simulink model "Two_Zone_MVDC_PSolver_Thermal_R2020b"  (R2020b)
settings: Solver=FixedStepDiscrete  StartTime=0.0  StopTime=30  FixedStep=TsELEC  RelTol=1e-3  EnableMultiTasking=on
InitFcn:
  | TsELEC = 25e-6;
  | Ts = 25e-6;
  | TsTHERMAL = 1e-3;
  | TsCont = TsELEC;
  | Rsnub = 1e4;
undefined symbols (not defined in the file or in its folder): DiscIntNeverNeededParam, ee_sli_rtmsupport, GABDA, GABDB, GBBDA, GBBDB, gcbh, GPMMA, GPPMB, GPPMC, SADA, SADB, SADC, SADD, SBDA, SBDB, SBDC, SCDA, SCDB, SCDC, SCDD, SDDA, SDDB, SDDC, SDDD, SDDE
libraries: fl_lib x201, nesl_utility x93, ee_lib x52, SimscapeFluids_lib x4, simulink x3, pid_lib x3, eeTransforms x3, sps_avr x2, powerlib_meascontrol x2, slrealtimetgmanagement x1
(part 5 of 5)

== system Two_Zone_MVDC_PSolver_Thermal_R2020b/Subsystem3/Control/Torque Control/Control_System/Current_Controllers/PI_Controller_Id ==
  I_ref : Inport
  I_fb : Inport  Port=2
  Constant : Constant  Value=0  SampleTime=TsELEC
  Discrete PID Controller : pid_lib/PID Controller  Controller=PID  Form=Parallel  TimeDomain=Discrete-time  UseExternalTs=off  SampleTime=TsELEC  IntegratorMethod=Forward Euler  FilterMethod=Forward Euler  ControllerParametersSource=internal  P=2/10  I=340/10  D=0  UseFilter=on  N=100  TunerSelectOption=Transfer Function Based (PID Tuner App)  InitialConditionSource=internal  InitialConditionForIntegrator=0  InitialConditionForFilter=0  DifferentiatorICPrevScaledInput=0  ExternalReset=either  TrackingMode=off  Kt=1  LimitOutput=off  SatLimitsSource=internal  UpperSaturationLimit=inf  LowerSaturationLimit=-inf  LinearizeAsGain=off  AntiWindupMode=none  Kb=1  POutMin=[]  POutMax=[]  IOutMin=[]  IOutMax=[]  DOutMin=[]  DOutMax=[]  NOutMin=[]  NOutMax=[]  SumOutMin=[]  SumOutMax=[]  SaturationOutMin=[]  SaturationOutMax=[]  PParamMin=[]  PParamMax=[]  IParamMin=[]  IParamMax=[]  DParamMin=[]  DParamMax=[]  NParamMin=[]  NParamMax=[]  KbParamMin=[]  KbParamMax=[]  KtParamMin=[]  KtParamMax=[]  KbOutMin=[]  KbOutMax=[]  KtOutMin=[]  KtOutMax=[]  IntegratorOutMin=[]  IntegratorOutMax=[]  FilterOutMin=[]  FilterOutMax=[]  SumI1OutMin=[]  SumI1OutMax=[]  SumI2OutMin=[]  SumI2OutMax=[]  SumI3OutMin=[]  SumI3OutMax=[]  SumI4OutMin=[]  SumI4OutMax=[]  SumDOutMin=[]  SumDOutMax=[]  DifferentiatorOutMin=[]  DifferentiatorOutMax=[]  FilterDiffOutCoefMin=[]  FilterDiffOutCoefMax=[]  ReciprocalOutMin=[]  ReciprocalOutMax=[]  SumDenOutMin=[]  SumDenOutMax=[]  SumNumOutMin=[]  SumNumOutMax=[]  DivideOutMin=[]  DivideOutMax=[]  UdiffTsProdOutMin=[]  UdiffTsProdOutMax=[]  NTsProdOutMin=[]  NTsProdOutMax=[]  UintegralTsProdOutMin=[]  UintegralTsProdOutMax=[]  UngainTsProdOutMin=[]  UngainTsProdOutMax=[]  IntegratorContinuousStateAttributes=''  IntegratorStateMustResolveToSignalObject=off  IntegratorRTWStateStorageClass=Auto  FilterContinuousStateAttributes=''  FilterStateMustResolveToSignalObject=off  FilterRTWStateStorageClass=Auto  ParallelPVariant=InternalParameters  IdealPVariant=Disabled  IVariant=InternalParameters  DVariant=InternalParameters  IntegratorVariant=Discrete  SatVariant=Disabled  AWVariant=Passthrough  PCopyVariant=Disabled  TRVariant=Disabled  FdbkBlocksVariant=Forward  IdealPFdbkVariant=Disabled  SatFdbkVariant=Disabled  DerivativeFilterVariant=ForwardEulerFilter  NVariant=InternalParameters  NCopyVariant=Disabled  FilterICVariant=InternalICsFilter  IntegratorICVariant=InternalICs  ExternalResetVariant=ExternalReset  TRSumVariant=Passthrough  SumFdbkVariant=Disabled  SumVariant=Sum_PID  TsampFilterVariant=InternalTs  TsampNgainVariant=Passthrough  TsampIntegralVariant=Passthrough  ExternalSaturationOutDataTypeStr=Inherit: Same as second input
  Sum : Sum  Inputs=|+-  OutDataTypeStr=Inherit: Same as first input
  V_ref : Outport  VectorParamsAs1DForOutWhenUnconnected=off
  wires:
  Constant/1 -> Discrete PID Controller/2
  Sum/1 -> Discrete PID Controller/1
  Discrete PID Controller/1 -> V_ref/1
  I_fb/1 -> Sum/2
  I_ref/1 -> Sum/1

== system Two_Zone_MVDC_PSolver_Thermal_R2020b/Subsystem3/Control/Torque Control/Control_System/Current_Controllers/PI_Controller_Iq ==
  I_ref : Inport
  I_fb : Inport  Port=2
  Constant : Constant  Value=0  SampleTime=TsELEC
  Discrete PID Controller : pid_lib/PID Controller  Controller=PID  Form=Parallel  TimeDomain=Discrete-time  UseExternalTs=off  SampleTime=TsELEC  IntegratorMethod=Forward Euler  FilterMethod=Forward Euler  ControllerParametersSource=internal  P=2/10  I=340/10  D=0  UseFilter=on  N=100  TunerSelectOption=Transfer Function Based (PID Tuner App)  InitialConditionSource=internal  InitialConditionForIntegrator=0  InitialConditionForFilter=0  DifferentiatorICPrevScaledInput=0  ExternalReset=either  TrackingMode=off  Kt=1  LimitOutput=off  SatLimitsSource=internal  UpperSaturationLimit=inf  LowerSaturationLimit=-inf  LinearizeAsGain=off  AntiWindupMode=none  Kb=1  POutMin=[]  POutMax=[]  IOutMin=[]  IOutMax=[]  DOutMin=[]  DOutMax=[]  NOutMin=[]  NOutMax=[]  SumOutMin=[]  SumOutMax=[]  SaturationOutMin=[]  SaturationOutMax=[]  PParamMin=[]  PParamMax=[]  IParamMin=[]  IParamMax=[]  DParamMin=[]  DParamMax=[]  NParamMin=[]  NParamMax=[]  KbParamMin=[]  KbParamMax=[]  KtParamMin=[]  KtParamMax=[]  KbOutMin=[]  KbOutMax=[]  KtOutMin=[]  KtOutMax=[]  IntegratorOutMin=[]  IntegratorOutMax=[]  FilterOutMin=[]  FilterOutMax=[]  SumI1OutMin=[]  SumI1OutMax=[]  SumI2OutMin=[]  SumI2OutMax=[]  SumI3OutMin=[]  SumI3OutMax=[]  SumI4OutMin=[]  SumI4OutMax=[]  SumDOutMin=[]  SumDOutMax=[]  DifferentiatorOutMin=[]  DifferentiatorOutMax=[]  FilterDiffOutCoefMin=[]  FilterDiffOutCoefMax=[]  ReciprocalOutMin=[]  ReciprocalOutMax=[]  SumDenOutMin=[]  SumDenOutMax=[]  SumNumOutMin=[]  SumNumOutMax=[]  DivideOutMin=[]  DivideOutMax=[]  UdiffTsProdOutMin=[]  UdiffTsProdOutMax=[]  NTsProdOutMin=[]  NTsProdOutMax=[]  UintegralTsProdOutMin=[]  UintegralTsProdOutMax=[]  UngainTsProdOutMin=[]  UngainTsProdOutMax=[]  IntegratorContinuousStateAttributes=''  IntegratorStateMustResolveToSignalObject=off  IntegratorRTWStateStorageClass=Auto  FilterContinuousStateAttributes=''  FilterStateMustResolveToSignalObject=off  FilterRTWStateStorageClass=Auto  ParallelPVariant=InternalParameters  IdealPVariant=Disabled  IVariant=InternalParameters  DVariant=InternalParameters  IntegratorVariant=Discrete  SatVariant=Disabled  AWVariant=Passthrough  PCopyVariant=Disabled  TRVariant=Disabled  FdbkBlocksVariant=Forward  IdealPFdbkVariant=Disabled  SatFdbkVariant=Disabled  DerivativeFilterVariant=ForwardEulerFilter  NVariant=InternalParameters  NCopyVariant=Disabled  FilterICVariant=InternalICsFilter  IntegratorICVariant=InternalICs  ExternalResetVariant=ExternalReset  TRSumVariant=Passthrough  SumFdbkVariant=Disabled  SumVariant=Sum_PID  TsampFilterVariant=InternalTs  TsampNgainVariant=Passthrough  TsampIntegralVariant=Passthrough  ExternalSaturationOutDataTypeStr=Inherit: Same as second input
  Sum : Sum  Inputs=|+-  OutDataTypeStr=Inherit: Same as first input
  V_ref : Outport  VectorParamsAs1DForOutWhenUnconnected=off
  wires:
  Constant/1 -> Discrete PID Controller/2
  Sum/1 -> Discrete PID Controller/1
  I_ref/1 -> Sum/1
  I_fb/1 -> Sum/2
  Discrete PID Controller/1 -> V_ref/1

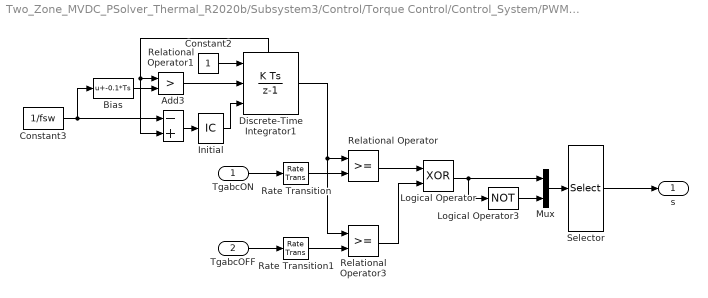
== system Two_Zone_MVDC_PSolver_Thermal_R2020b/Subsystem3/Control/Torque Control/Control_System/PWM Generator (Three-phase, Two-level)/Gate Signal Generator ==
  TgabcON : Inport
  TgabcOFF : Inport  Port=2
  Add3 : Sum  Inputs=-+
  Bias : Bias  Bias=-0.1*Ts
  Constant2 : Constant
  Constant3 : Constant  Value=1/fsw
  Discrete-Time Integrator1 : DiscreteIntegrator  ExternalReset=rising  InitialConditionSource=external  SampleTime=Ts  ShowStatePort=on  ICPrevOutput=DiscIntNeverNeededParam  ICPrevScaledInput=DiscIntNeverNeededParam
  Initial : InitialCondition  Value=GateGeneratorX0
  Logical Operator : Logic  Operator=XOR  AllPortsSameDT=off  OutDataTypeStr=boolean
  Logical Operator3 : Logic  Operator=NOT  AllPortsSameDT=off  OutDataTypeStr=boolean
  Mux : Mux  Inputs=2
  Rate Transition : RateTransition  Deterministic=off
  Rate Transition1 : RateTransition  Deterministic=off
  Relational Operator : RelationalOperator  OutDataTypeStr=boolean  RndMeth=Nearest
  Relational Operator1 : RelationalOperator  Operator=>  OutDataTypeStr=boolean  RndMeth=Nearest
  Relational Operator3 : RelationalOperator  OutDataTypeStr=boolean  RndMeth=Nearest
  Selector : Selector  InputPortWidth=6  IndexOptions=Index vector (dialog)  Indices=[1 4 2 5 3 6]  OutputSizes=1
  s : Outport  VectorParamsAs1DForOutWhenUnconnected=off
  wires:
  Rate Transition1/1 -> Relational Operator3/2
  Rate Transition/1 -> Relational Operator/2
  TgabcOFF/1 -> Rate Transition1/1
  TgabcON/1 -> Rate Transition/1
  Constant3/1 -> Add3/1, Bias/1
  Discrete-Time Integrator1/State -> Relational Operator1/1, Add3/2
  Constant2/1 -> Discrete-Time Integrator1/1
  Initial/1 -> Discrete-Time Integrator1/3
  Add3/1 -> Initial/1
  Relational Operator1/1 -> Discrete-Time Integrator1/2
  Bias/1 -> Relational Operator1/2
  Discrete-Time Integrator1/1 -> Relational Operator/1, Relational Operator3/1
  Selector/1 -> s/1
  Mux/1 -> Selector/1
  Logical Operator3/1 -> Mux/2
  Logical Operator/1 -> Mux/1, Logical Operator3/1
  Relational Operator/1 -> Logical Operator/1
  Relational Operator3/1 -> Logical Operator/2

== matlab function Two_Zone_MVDC_PSolver_Thermal_R2020b/Subsystem3/Control/Torque Control/Control_System/PWM Generator (Three-phase, Two-level)/Switching Time Calculation ==
  settings: sampleTime=1
  data: Vabc input; TgabcON output; vdc input; TgabcOFF output; ModWave output; fsw parameter; PWM parameter
function [TgabcON,TgabcOFF,ModWave]  = switchingTime(Vabc,vdc,fsw,PWM)

[TgabcON,TgabcOFF,ModWave] = ee.control.pwmSwitchingTimeTwoLevel(Vabc,vdc,fsw,PWM);
